simulink model "Assignment_3_solution"  (R2019b)
settings: Solver=ode23t  StartTime=0.0  StopTime=10  MaxStep=0.1  RelTol=1e-3
libraries: powerlib x13, powerlib_meascontrol x3
settings Model: Creator=andreasthingvad  LastModifiedBy=matm
settings SolverCC: ShapePreserveControl=EnableAll  SolverResetMethod=Robust

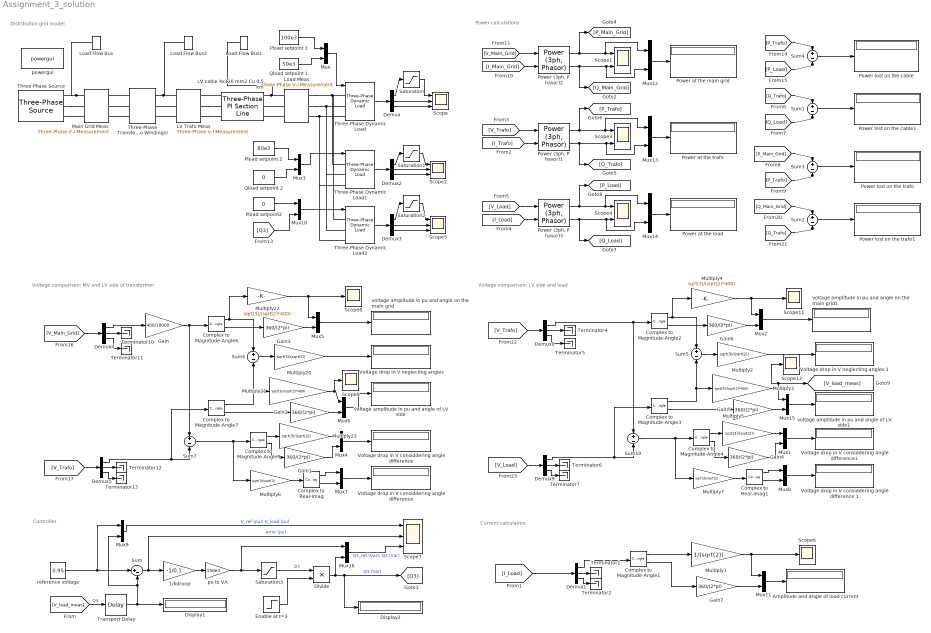
== system Assignment_3_solution ==
  note: Distribution grid model
  note: Current calculation
  note: Controller
  note: Voltage comparison: LV side and load
  note: Voltage comparison: MV and LV side of transformer
  note: Power calculations
  1/kdroop : Gain  Gain=-1/0.1
  Amplitude and angle of load current : Display
      settings: Decimation=3
  Complex to Magnitude-Angle{1..4,6..8} (7 alike) : ComplexToMagnitudeAngle
  Complex to Real-Imag : ComplexToRealImag
  Complex to Real-Imag1 : ComplexToRealImag
  Demux{,1..5,8..9} (8 alike) : Demux  Outputs=3
  Display1 : Display
      settings: Decimation=3
  Display2 : Display
      settings: Decimation=3
  Divide : Product  Inputs=**
  Enable at t=3 : Step  Time=3  SampleTime=0
  Gain : Gain  Gain=400/10000
  Gain{1..7} (7 alike) : Gain  Gain=360/(2*pi)
  LV Trafo Meas : powerlib/Measurements/Three-Phase V-I Measurement  VoltageMeasurement=phase-to-ground  SetLabelV=on  LabelV=V_Trafo  Vpu=off  VpuLL=off  CurrentMeasurement=yes  SetLabelI=on  LabelI=I_Trafo  Ipu=off  Pbase=100e6  Vbase=500e3  OutputType=Complex  PhasorSimulation=on  PSBequivalent=0
  LV cable 4x120 mm2 Cu 0.5 km : powerlib/Elements/Three-Phase PI Section Line  LConnTagsString=a|b|c  RConnTagsString=A|B|C  Frequency=50  Resistances=[0.1556 0.6224]  Inductances=[0.00023 0.0009172]  Capacitances=[0.92e-6 0.485e-6]  Length=0.5
  Load Flow Bus : powerlib/Measurements/Load Flow Bus  LConnTagsString=a  Phases=single  Connectors=on one side  ID=Slack  Vbase=10e3  Vref=1  Vangle=0  VLF=1  VLFb=1  VLFc=1  angleLF=0  angleLFb=0  angleLFc=0
  Load Flow Bus1 : powerlib/Measurements/Load Flow Bus  LConnTagsString=a  Phases=single  Connectors=on one side  ID=Load  Vbase=400  Vref=1  Vangle=0  VLF=0.923  VLFb=1  VLFc=1  angleLF=-2.499  angleLFb=0  angleLFc=0
  Load Flow Bus2 : powerlib/Measurements/Load Flow Bus  LConnTagsString=a  Phases=single  Connectors=on one side  ID=Trafo LV  Vbase=0.4e3  Vref=1  Vangle=0  VLF=0.9972  VLFb=1  VLFc=1  angleLF=-0.5339  angleLFb=0  angleLFc=0
  Load Meas : powerlib/Measurements/Three-Phase V-I Measurement  VoltageMeasurement=phase-to-ground  SetLabelV=on  LabelV=V_Load  Vpu=off  VpuLL=off  CurrentMeasurement=yes  SetLabelI=on  LabelI=I_Load  Ipu=off  Pbase=100e6  Vbase=500e3  OutputType=Complex  PhasorSimulation=on  PSBequivalent=0
  Main Grid Meas : powerlib/Measurements/Three-Phase V-I Measurement  VoltageMeasurement=phase-to-ground  SetLabelV=on  LabelV=V_Main_Grid  Vpu=off  VpuLL=off  CurrentMeasurement=yes  SetLabelI=on  LabelI=I_Main_Grid  Ipu=off  Pbase=100e6  Vbase=500e3  OutputType=Complex  PhasorSimulation=on  PSBequivalent=0
  Multiply1 : Gain  Gain=1/(sqrt(2))
  Multiply{2,5,20,23} (4 alike) : Gain  Gain=sqrt(3)/(sqrt(2))
  Multiply{3..4,21..22} (4 alike) : Gain  Gain=sqrt(3)/(sqrt(2)*400)
  Multiply6 : Gain  Gain=sqrt(3)/sqrt(2)
  Multiply7 : Gain  Gain=sqrt(3)/sqrt(2)
  Mux{,1..16} (17 alike) : Mux  Inputs=2
  Pload setpoint 1 : Constant  Value=100e3
  Pload setpoint 2 : Constant  Value=80e3
  Pload setpoint2 : Constant  Value=0
  "Power (3ph, P hasor)1" : powerlib_meascontrol/Measurements/Power (3ph, Phasor)
      settings: SourceProductBaseCode=PS
  "Power (3ph, P hasor)2" : powerlib_meascontrol/Measurements/Power (3ph, Phasor)
      settings: SourceProductBaseCode=PS
  "Power (3ph, P hasor)3" : powerlib_meascontrol/Measurements/Power (3ph, Phasor)
      settings: SourceProductBaseCode=PS
  Power at the load : Display
      settings: Decimation=3
  Power at the main grid : Display
      settings: Decimation=3
  Power at the trafo : Display
      settings: Decimation=3
  Power lost on the cable : Display
      settings: Decimation=3
  Power lost on the cable1 : Display
      settings: Decimation=3
  Power lost on the trafo : Display
      settings: Decimation=3
  Power lost on the trafo1 : Display
      settings: Decimation=3
  Qload setpoint 1 : Constant  Value=50e3
  Qload setpoint 2 : Constant  Value=0
  Saturation : Saturate  UpperLimit=1.15  LowerLimit=0.85
  Saturation1 : Saturate  UpperLimit=1.15  LowerLimit=0.85
  Saturation2 : Saturate  UpperLimit=1.15  LowerLimit=0.85
  Saturation3 : Saturate  UpperLimit=150e3  LowerLimit=-150e3
  Scope{,2,5,7} (4 alike) : Scope  NumInputPorts=3
  Scope1 : Scope  NumInputPorts=2
  Scope{6,8..9,11..12} (5 alike) : Scope
  Scope3 : Scope  NumInputPorts=2
  Scope4 : Scope  NumInputPorts=2
  Sum : Sum  Inputs=|+-
  Sum{1..7,10} (8 alike) : Sum  Inputs=+-
  Terminator{1..2,4..7,10..13} (10 alike) : Terminator
  Three-Phase Dynamic Load : powerlib/Elements/Three-Phase Dynamic Load  NominalVoltage=[ 0.4e3 50 ]  ActiveReactivePowers=[100000 50e3]  PositiveSequence=[0.922978 -2.49938]  ExternalControl=on  NpNq=[1.3 2]  TimeConstants="[0  0  0  0]"  MinimumVoltage=0.7  Tfilter=1e-4  LoadFlowParameters=[4,0,0,0,0]
      settings: SourceProductBaseCode=PS
  Three-Phase Dynamic Load1 : powerlib/Elements/Three-Phase Dynamic Load  NominalVoltage=[ 0.4e3 50 ]  ActiveReactivePowers=[80000 0]  PositiveSequence=[0.922978 -2.49938]  ExternalControl=on  NpNq=[1.3 2]  TimeConstants="[0  0  0  0]"  MinimumVoltage=0.7  Tfilter=1e-4  LoadFlowParameters=[4,0,0,0,0]
      settings: SourceProductBaseCode=PS
  Three-Phase Dynamic Load2 : powerlib/Elements/Three-Phase Dynamic Load  NominalVoltage=[ 0.4e3 50 ]  ActiveReactivePowers=[0 0]  PositiveSequence=[0.922978 -2.49938]  ExternalControl=on  NpNq=[1.3 2]  TimeConstants="[0  0  0  0]"  MinimumVoltage=0.7  Tfilter=1e-4  LoadFlowParameters=[4,0,0,0,0]
      settings: SourceProductBaseCode=PS
  Three-Phase Transformer (Two Windings) : powerlib/Elements/Three-Phase Transformer (Two Windings)  Winding1Connection=Yg  Winding2Connection=Yg  CoreType=Three single-phase transformers  SetSaturation=off  Hysteresis=off  DataFile='hysteresis'  SetInitialFlux=off  Measurements=None  UNITS=pu  NominalPower=[ 630e3 , 50 ]  Winding1=[ 10e3 , 0.005 , 0.0195 ]  Winding2=[ 0.4e3 , 0.005 , 0.0195]  Rm=500  Lm=500  L0=0.5  Saturation=[ 0,0 ; 0.0024,1.2 ; 1.0,1.52 ]  InitialFluxes=[ 0.8 , -0.8 , 0.7 ]  BreakLoop=off  DiscreteSolver=Trapezoidal iterative  DataType=off  TransfoNumber=1
  Three-Phase Source : powerlib/Electrical Sources/Three-Phase Source  InternalConnection=Yg  VoltagePhases=off  Voltage=(10000)*1.00046  PhaseAngle=0.17385  Voltage_phases=[25e3 25e3 25e3]/sqrt(3)  PhaseAngles_phases=[0 -120 +120]  Frequency=50  NonIdealSource=on  SpecifyImpedance=on  Resistance=10e6  Inductance=0.4e-3  ShortCircuitLevel=50e6  BaseVoltage=10e3  XRratio=10  BusType=swing  Pref=10e3  Qref=0  Prefabc=[10e3, 10e3, 10e3]  Qrefabc=[0, 0, 0]  Qmin=-inf  Qmax=inf
  Transport Delay : TransportDelay  DelayTime=0.5  InitialOutput=0.95
  Voltage drop in V considdering angle difference : Display
      settings: Decimation=3
  "Voltage drop in V considdering angle difference " : Display
      settings: Decimation=3
  Voltage drop in V considdering angle difference 1 : Display
      settings: Decimation=3
  Voltage drop in V considdering angle difference1 : Display
      settings: Decimation=3
  "Voltage drop in V neglecting angles " : Display
      settings: Decimation=3
  Voltage drop in V neglecting angles 1 : Display
      settings: Decimation=3
  powergui : powerlib/powergui  Priority=1  SimulationMode=Phasor  SampleTime=50e-6  frequency=50  Iterations=50  frequencyindice=50  Pbase=1e6  ErrMax=0.001  UnitsV=kV  UnitsW=kW  buscounter=0  FunctionMessages=off  echomessages=off  EnableUseOfTLC=off  CurrentSourceSwitches=off  DisableSnubberDevices=off  DisableRonSwitches=off  DisableVfSwitches=off  DisplayEquations=off  AutomaticDiscreteSolvers=off  SolverType=Tustin/Backward Euler (TBE)  Interpol=off  ExternalGateDelay=off  methode=off  Ts=100  x0status=blocks  SPID=on  SwTol=0  HookPort=off  NonlinearTolerance=1e-4  nMaxIteration=100  ContinueOnMaxIteration=off  RestoreLinks=warning  ResistiveCurrentMeasurement=off  Frange=[0:2:500]  Ylog=off  Xlog=on  ShowGrid=off  save=off  variable=ZData  structure=0  ZoomFFT=off  StartTime=0.0  cycles=1  DisplayStyle=1  fundamental=60  FreqAxis=off  MaxFrequency=1000  frequencyindicesteady=1  RmsSteady=1  display=off
      settings: SourceProductName=Simscape Electrical
  pu to VA : Gain  Gain=150e3
  reference voltage : Constant  Value=0.95
  voltage amplitude in pu and angle of LV side : Display
      settings: Decimation=3
  voltage amplitude in pu and angle of LV side1 : Display
      settings: Decimation=3
  voltage amplitude in pu and angle on the main grid : Display
      settings: Decimation=3
  voltage amplitude in pu and angle on the main grid1 : Display
      settings: Decimation=3
  wires:
  "Power (3ph, P hasor)2"/1 -> Mux12/1, Scope1/1, [P_Main_Grid]
  [I_Load] -> Demux1/1
  Mux5/1 -> voltage amplitude in pu and angle on the main grid/1
  Sum/1 -> Scope7/2, 1/kdroop/1  "error (pu)"
  Complex to Magnitude-Angle7/2 -> Gain2/1
  Mux/1 -> Three-Phase Dynamic Load/1
  Demux/2 -> Scope/2
  Three-Phase Dynamic Load2/1 -> Demux3/1
  Mux6/1 -> voltage amplitude in pu and angle of LV side/1
  Complex to Magnitude-Angle6/1 -> Sum6/1, Multiply22/1
  Pload setpoint 2/1 -> Mux3/1
  Demux3/2 -> Scope5/2
  Multiply22/1 -> Scope8/1, Mux5/1
  Multiply21/1 -> Scope9/1, Mux6/1
  Demux5/2 -> Terminator12/1
  [I_Main_Grid] -> "Power (3ph, P hasor)2"/2
  Sum7/1 -> Multiply6/1, Complex to Magnitude-Angle8/1
  Mux4/1 -> Voltage drop in V considdering angle difference/1
  Mux10/1 -> Three-Phase Dynamic Load2/1
  Saturation/1 -> Scope/1
  Gain/1 -> Complex to Magnitude-Angle6/1, Sum7/1
  Complex to Magnitude-Angle6/2 -> Gain3/1
  [V_Trafo] -> Demux5/1
  [V_Main_Grid] -> Demux4/1
  Pload setpoint 1/1 -> Mux/1
  Complex to Magnitude-Angle7/1 -> Sum6/2, Multiply21/1
  Demux/3 -> Scope/3
  Three-Phase Dynamic Load/1 -> Demux/1
  Demux4/3 -> Terminator11/1
  Sum6/1 -> Multiply20/1
  [V_Main_Grid] -> "Power (3ph, P hasor)2"/1
  Multiply20/1 -> "Voltage drop in V neglecting angles "/1
  Complex to Magnitude-Angle8/2 -> Gain1/1
  Demux5/3 -> Terminator13/1
  Demux4/2 -> Terminator10/1
  Demux5/1 -> Complex to Magnitude-Angle7/1, Sum7/2
  Demux2/3 -> Scope2/3
  Complex to Magnitude-Angle8/1 -> Multiply23/1
  Demux4/1 -> Gain/1
  Demux/1 -> Saturation/1
  Demux3/3 -> Scope5/3
  Complex to Magnitude-Angle1/1 -> Multiply1/1
  Multiply23/1 -> Mux4/1
  Mux11/1 -> Amplitude and angle of load current/1
  Demux1/3 -> Terminator2/1
  Demux1/2 -> Terminator1/1
  Demux1/1 -> Complex to Magnitude-Angle1/1
  Qload setpoint 2/1 -> Mux3/2
  Mux3/1 -> Three-Phase Dynamic Load1/1
  Demux3/1 -> Saturation2/1
  Saturation1/1 -> Scope2/1
  Saturation2/1 -> Scope5/1
  Demux2/1 -> Saturation1/1
  Multiply1/1 -> Mux11/1, Scope6/1
  Demux2/2 -> Scope2/2
  Pload setpoint2/1 -> Mux10/1
  "Power (3ph, P hasor)2"/2 -> [Q_Main_Grid], Mux12/2, Scope1/2
  Complex to Magnitude-Angle1/2 -> Gain7/1
  Three-Phase Dynamic Load1/1 -> Demux2/1
  reference voltage/1 -> Mux9/1, Sum/1
  Transport Delay/1 -> Display1/1, Mux9/2, Sum/2
  1/kdroop/1 -> pu to VA/1
  Enable at t=3/1 -> Divide/2
  pu to VA/1 -> Mux16/1, Saturation3/1
  Mux12/1 -> Power at the main grid/1
  Mux13/1 -> Power at the trafo/1
  "Power (3ph, P hasor)1"/2 -> Scope3/2, Mux13/2, [Q_Trafo]
  [V_Trafo] -> "Power (3ph, P hasor)1"/1
  [I_Trafo] -> "Power (3ph, P hasor)1"/2
  "Power (3ph, P hasor)1"/1 -> [P_Trafo], Scope3/1, Mux13/1
  "Power (3ph, P hasor)3"/1 -> Mux14/1, Scope4/1, [P_Load]
  [I_Load] -> "Power (3ph, P hasor)3"/2
  [V_Load] -> "Power (3ph, P hasor)3"/1
  "Power (3ph, P hasor)3"/2 -> [Q_Load], Mux14/2, Scope4/2
  Mux14/1 -> Power at the load/1
  Sum4/1 -> Power lost on the cable/1
  [P_Load] -> Sum4/2
  [P_Trafo] -> Sum4/1
  [Q_Trafo] -> Sum1/1
  [Q_Load] -> Sum1/2
  Sum1/1 -> Power lost on the cable1/1
  Sum2/1 -> Power lost on the trafo1/1
  [Q_Trafo] -> Sum2/2
  [Q_Main_Grid] -> Sum2/1
  [P_Main_Grid] -> Sum3/1
  [P_Trafo] -> Sum3/2
  Sum3/1 -> Power lost on the trafo/1
  [V_load_meas] -> Transport Delay/1  "Q3"
  Divide/1 -> Display2/1, [Q3], Mux16/2  "Q3 (Var)"
  Gain2/1 -> Mux6/2
  Gain1/1 -> Mux4/2
  Multiply2/1 -> Voltage drop in V neglecting angles 1/1
  Complex to Magnitude-Angle2/2 -> Gain6/1
  Complex to Magnitude-Angle4/1 -> Multiply5/1
  Demux8/2 -> Terminator4/1
  Sum5/1 -> Multiply2/1
  Complex to Magnitude-Angle2/1 -> Sum5/1, Multiply4/1
  Demux9/3 -> Terminator7/1
  Complex to Magnitude-Angle4/2 -> Gain4/1
  Demux9/1 -> Complex to Magnitude-Angle3/1, Sum10/2
  Multiply5/1 -> Mux1/1
  Demux8/3 -> Terminator5/1
  Mux1/1 -> Voltage drop in V considdering angle difference1/1
  Mux15/1 -> voltage amplitude in pu and angle of LV side1/1
  Complex to Magnitude-Angle3/2 -> Gain5/1
  Complex to Magnitude-Angle3/1 -> Sum5/2, Multiply3/1
  [V_Trafo] -> Demux8/1
  [V_Load] -> Demux9/1
  Multiply3/1 -> Mux15/1, Scope12/1, [V_load_meas]
  Demux9/2 -> Terminator6/1
  Gain4/1 -> Mux1/2
  Multiply4/1 -> Scope11/1, Mux2/1
  Gain5/1 -> Mux15/2
  Mux2/1 -> voltage amplitude in pu and angle on the main grid1/1
  Demux8/1 -> Sum10/1, Complex to Magnitude-Angle2/1
  Gain3/1 -> Mux5/2
  Gain6/1 -> Mux2/2
  Saturation3/1 -> Divide/1  "Q3"
  Complex to Real-Imag/1 -> Mux7/1
  Complex to Real-Imag/2 -> Mux7/2
  Mux7/1 -> "Voltage drop in V considdering angle difference "/1
  Multiply6/1 -> Complex to Real-Imag/1
  Complex to Real-Imag1/2 -> Mux8/2
  Multiply7/1 -> Complex to Real-Imag1/1
  Complex to Real-Imag1/1 -> Mux8/1
  Sum10/1 -> Multiply7/1, Complex to Magnitude-Angle4/1
  Mux8/1 -> Voltage drop in V considdering angle difference 1/1
  Gain7/1 -> Mux11/2
  Mux9/1 -> Scope7/1  "V_ref (pu); V_load (pu)"
  Mux16/1 -> Scope7/3  "Q3_ref (Var); Q3 (Var)"
  [Q3] -> Mux10/2
  Qload setpoint 1/1 -> Mux/2
  connections:
  LV cable 4x120 mm2 Cu 0.5 km/RConn1 -- Load Meas/LConn1 -- Load Flow Bus1/LConn1
  Main Grid Meas/LConn1 -- Three-Phase Source/RConn1 -- Load Flow Bus/LConn1
  Three-Phase Transformer (Two Windings)/RConn1 -- LV Trafo Meas/LConn1 -- Load Flow Bus2/LConn1
  Load Meas/RConn1 -- Three-Phase Dynamic Load2/LConn1 -- Three-Phase Dynamic Load1/LConn1 -- Three-Phase Dynamic Load/LConn1
  Load Meas/RConn2 -- Three-Phase Dynamic Load2/LConn2 -- Three-Phase Dynamic Load1/LConn2 -- Three-Phase Dynamic Load/LConn2
  Load Meas/RConn3 -- Three-Phase Dynamic Load2/LConn3 -- Three-Phase Dynamic Load1/LConn3 -- Three-Phase Dynamic Load/LConn3
  Load Meas/LConn2 -- LV cable 4x120 mm2 Cu 0.5 km/RConn2
  Load Meas/LConn3 -- LV cable 4x120 mm2 Cu 0.5 km/RConn3
  Three-Phase Transformer (Two Windings)/LConn1 -- Main Grid Meas/RConn1
  Three-Phase Source/RConn2 -- Main Grid Meas/LConn2
  Three-Phase Transformer (Two Windings)/LConn2 -- Main Grid Meas/RConn2
  Three-Phase Source/RConn3 -- Main Grid Meas/LConn3
  LV Trafo Meas/RConn3 -- LV cable 4x120 mm2 Cu 0.5 km/LConn3
  Main Grid Meas/RConn3 -- Three-Phase Transformer (Two Windings)/LConn3
  LV Trafo Meas/LConn2 -- Three-Phase Transformer (Two Windings)/RConn2
  LV Trafo Meas/LConn3 -- Three-Phase Transformer (Two Windings)/RConn3
  LV cable 4x120 mm2 Cu 0.5 km/LConn1 -- LV Trafo Meas/RConn1
  LV Trafo Meas/RConn2 -- LV cable 4x120 mm2 Cu 0.5 km/LConn2
